simulink model "alfa_window_in_Ug"  (R2018b)
settings: Solver=VariableStepDiscrete  StartTime=0  StopTime=24*3600  MaxStep=1  RelTol=1e-3  EnableMultiTasking=on
libraries: carnot x5
settings Model: Creator=drhf  LastModifiedBy=drhf
settings DataIOCC: SaveFormat=Array  SignalLoggingSaveFormat=ModelDataLogs
settings OptimizationCC: ExpressionDepthLimit=2147483647  LifeSpan=inf
settings DebuggingCC: UnderspecifiedInitializationDetection=Classic  MergeDetectMultiDrivingBlocksExec=none  SolverPrmCheckMsg=warning  StateNameClashWarn=warning  SFUnexpectedBacktrackingDiag=warning  SFNoUnconditionalDefaultTransitionDiag=warning  SFExecutionAtInitializationDiag=none
settings HardwareCC: ProdBitPerPointer=32  ProdBitPerSizeT=32  ProdBitPerPtrDiffT=32  ProdLargestAtomicFloat=None  ProdIntDivRoundTo=Undefined  ProdEndianess=Unspecified  ProdWordSize=32  ProdHWDeviceType=32-bit Generic
settings ModelReferenceCC: PropagateSignalLabelsOutOfModel=off
settings SFSimCC: SimUseLocalCustomCode=off
settings RTWCC: RTWUseLocalCustomCode=off
settings CodeAppCC: StateflowObjectComments=on
settings GRTTargetCC: TargetLangStandard=C89/C90 (ANSI)  GeneratePreprocessorConditionals=Disable all  CombineOutputUpdateFcns=off  GRTInterface=on
settings ConfigComp: CovMetricSettings=dw  CovHtmlReporting=on  CovSaveCumulativeToWorkspaceVar=on  CovSaveSingleToWorkspaceVar=on  CovExternalEMLEnable=off

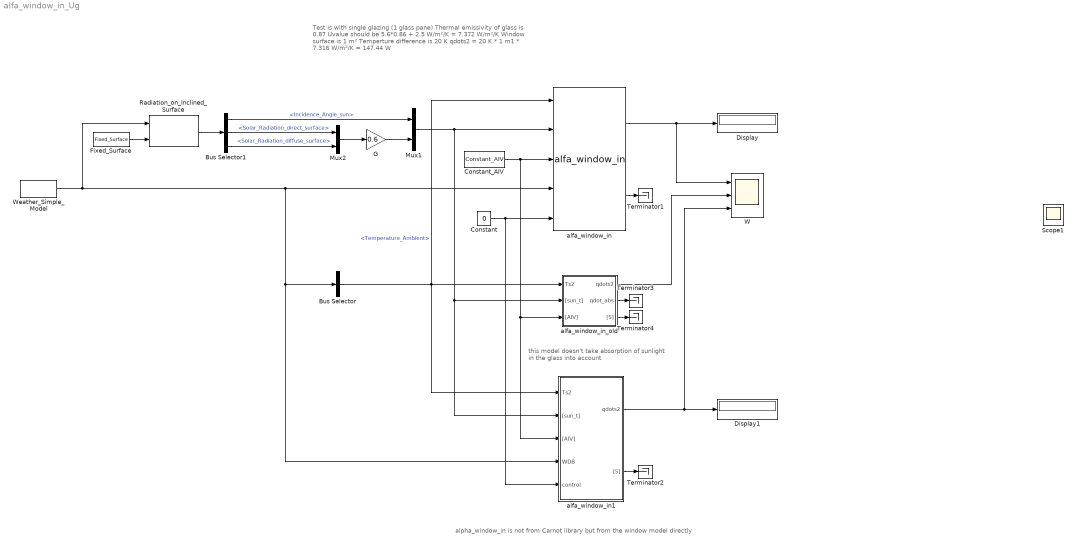
== system alfa_window_in_Ug ==
  note: this model doesn't take absorption
      | of sunlight in the glass into account
  note: Test is with single glazing (1 glass pane)
      | Thermal emissivity of glass is 0.87
      | Uvalue should be 5.6*0.86 + 2.5 W/m²/K = 7.372 W/m²/K
      | Window surface is 1 m²
      | Temperture difference is 20 K
      | qdots2 = 20 K * 1 m1 * 7.316 W/m²/K = 147.44 W
  note: alpha_window_in is not from Carnot library but from the window model directly
  Bus Selector : BusSelector  OutputSignals=Temperature_Ambient
  Bus Selector1 : BusSelector  OutputSignals=Incidence_Angle_sun,Solar_Radiation_direct_surface,Solar_Radiation_diffuse_surface
  Constant : Constant  Value=0
  Constant_AIV : carnot/Source/Ventilation/Constant_AIV  Tsens=20  Tcon=20  Trad=20  mw=0.012  mco=0.01  rhoair=1.2  cpair=1004  pair=100000  nair=0.5
      settings: SourceProductName=Carnot
  Display : Display
  Display1 : Display
  Fixed_Surface : carnot/Weather/Fixed_Surface  colangle=90  colazi=0  colrot=0
      settings: SourceProductName=Carnot
  G : Gain  Gain=0.6
  Mux1 : Mux  Inputs=2
  Mux2 : Mux  Inputs=2
  Radiation_on_Inclined_Surface : carnot/Weather/Radiation_on_Inclined_Surface  sky=Perez 1990  reflect=0.2
      settings: SourceProductName=Carnot
  Terminator{1..4} (4 alike) : Terminator
  W : Scope  NumInputPorts=3
  Weather_Simple_Model : carnot/Weather/Weather_Simple_Model  Ibn=900  Idg=100  tamb=0  deltaTsky=0  rh=50  precip="10e-3/24/3600           % 10 mm in 24 h"  cloud=0.125  p=1013e2  vw=0  wdir=270  lat=60  colangle=0  colazi=0  colrot=0
      settings: SourceProductName=Carnot
  alfa_window_in : carnot/Basic/Heat_Transfer/alfa_window_in  type_glazing=double glazing normal  gvalue=0.8  tauzero=0.9  emission_in=0.87  wallsurface=1  frame=0  numlayer=1  shad_type=No shading  tau_shad=0.01  bli_a=0.05  bli_b=1  bli_c=0.05  bli_d=0.05  bli_alpha=90  bli_refl=0.2
      settings: SourceProductName=Carnot
  alfa_window_in1 : Subsystem  mask(ALFA){}
      mask help:
      | Convective and radiative heat transfer at the INDOOR SURFACE OF A VERTICAL WINDOW with 1-4 layers (each 3 ... 8 mm thick).
      |
      | Ts  : temperature of window surface, °C,
      | [sun_t]  : sun data (incidence angle, direct and diffuse radiation
      |     at tilted window surface),
      | [AIV]  : conditions of zone node,
      | qdots  : specific heat flow into window construction, W/m^2,
      | [S]  : heat and air flow to zone node.
  alfa_window_in_old : Subsystem  mask(ALFA){gvalue=0.7, emission_in=0.87, wallsurface=1, frame=0.1, numlayer=2}
      mask prompts: gvalue "Energy transmission by sunlight (g-value) 0..1"; emission_in "Longwave emissivity (0..1)"; wallsurface "Surface of the window (with frame) in m²"; frame "Share of the frame on the surface (0...1)"; numlayer "Number of glass panes"
      mask help:
      | Convective and radiative heat transfer at the INDOOR SURFACE OF A VERTICAL WINDOW with 1-4 layers (each 3 ... 8 mm thick).
      |
      | Ts  : temperature of window surface, °C,
      | [sun_t]  : sun data (incidence angle, direct and diffuse radiation
      |     at tilted window surface),
      | [AIV]  : conditions of zone node,
      | qdots  : specific heat flow into window construction, W/m^2,
      | qdot_abs : specific irradiation absorption within window
      |     construction,  W/m^2,
      | [S]  : heat and air flow to zone node.
      mask Help: web(fullfile(path_carnot('help'),'alfa_window_in.html'),'-helpbrowser')
  Scope1 : Scope
  wires:
  alfa_window_in/1 -> Display/1, W/1
  Bus Selector/1 -> alfa_window_in/1, alfa_window_in1/1(Ts2), alfa_window_in_old/1(Ts2)  "<Temperature_Ambient>"
  Constant_AIV/1 -> alfa_window_in/3, alfa_window_in_old/3("[AIV]"), alfa_window_in1/3("[AIV]")
  Mux1/1 -> alfa_window_in1/2("[sun_t]"), alfa_window_in_old/2("[sun_t]"), alfa_window_in/2
  Weather_Simple_Model/1 -> Radiation_on_Inclined_Surface/1, Bus Selector/1, alfa_window_in1/4(WDB), alfa_window_in/4
  Constant/1 -> alfa_window_in1/5(control), alfa_window_in/5
  alfa_window_in_old/2(qdot_abs) -> Terminator3/1
  alfa_window_in_old/3("[S]") -> Terminator4/1
  alfa_window_in_old/1(qdots2) -> W/2
  Bus Selector1/1 -> Mux1/1  "<Incidence_Angle_sun>"
  Bus Selector1/3 -> Mux2/2  "<Solar_Radiation_diffuse_surface>"
  Radiation_on_Inclined_Surface/1 -> Bus Selector1/1
  Bus Selector1/2 -> Mux2/1  "<Solar_Radiation_direct_surface>"
  Mux2/1 -> G/1
  Fixed_Surface/1 -> Radiation_on_Inclined_Surface/2
  G/1 -> Mux1/2
  alfa_window_in/2 -> Terminator1/1
  alfa_window_in1/2("[S]") -> Terminator2/1
  alfa_window_in1/1(qdots2) -> Display1/1, W/3

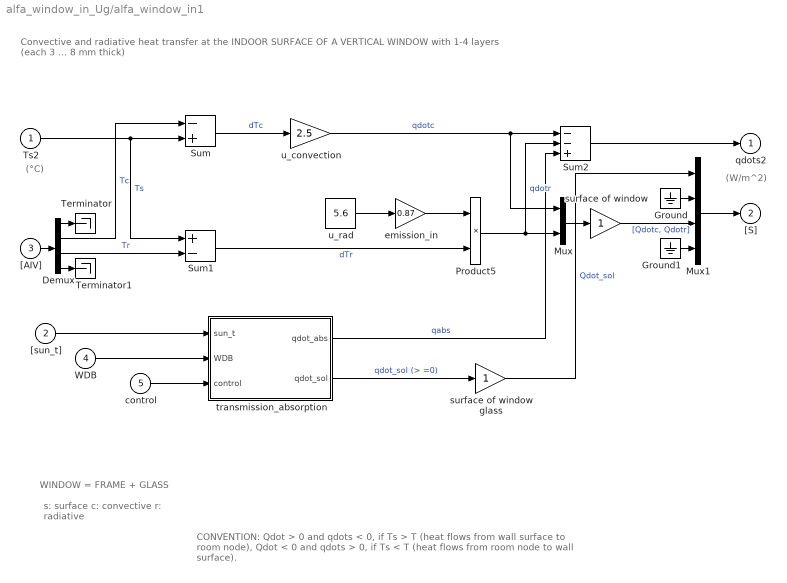
== system alfa_window_in_Ug/alfa_window_in1 ==
  note: (°C)
  note: Convective and radiative heat transfer at the INDOOR SURFACE OF A VERTICAL WINDOW
      | with 1-4 layers (each 3 ... 8 mm thick)
  note: WINDOW = FRAME + GLASS
  note: s: surface
      | c: convective
      | r: radiative
  note: CONVENTION:
      | Qdot > 0 and qdots < 0, if Ts > T (heat flows from wall surface to room node),
      | Qdot < 0 and qdots > 0, if Ts < T (heat flows from room node to wall surface).
  note: (W/m^2)
  Ts2 : Inport
  "[sun_t]" : Inport  Port=2
  "[AIV]" : Inport  Port=3
  WDB : Inport  Port=4
  control : Inport  Port=5
  Demux : Demux  Outputs=[1 1 1 6]
  Ground : Ground
  Ground1 : Ground
  Mux : Mux  Inputs=2
  Mux1 : Mux  Inputs=[1 5 2 5]
  Product5 : Product  SaturateOnIntegerOverflow=on  RndMeth=Zero  InputSameDT=on  OutDataTypeStr=Inherit: Same as first input
  Sum : Sum  Inputs=-+  SaturateOnIntegerOverflow=on  InputSameDT=on  OutDataTypeStr=Inherit: Same as first input
  Sum1 : Sum  Inputs=+-  SaturateOnIntegerOverflow=on  InputSameDT=on  OutDataTypeStr=Inherit: Same as first input
  Sum2 : Sum  Inputs=--+  SaturateOnIntegerOverflow=on  InputSameDT=on  OutDataTypeStr=Inherit: Same as first input
  Terminator : Terminator
  Terminator1 : Terminator
  emission_in : Gain  Gain=0.87  SaturateOnIntegerOverflow=on  OutDataTypeStr=Inherit: Same as input  ParamDataTypeStr=Inherit: Same as input
  surface of window : Gain  SaturateOnIntegerOverflow=on  OutDataTypeStr=Inherit: Same as input  ParamDataTypeStr=Inherit: Same as input
  surface of window glass : Gain  SaturateOnIntegerOverflow=on  OutDataTypeStr=Inherit: Same as input  ParamDataTypeStr=Inherit: Same as input
  transmission_absorption : Subsystem
  u_convection : Gain  Gain=2.5  SaturateOnIntegerOverflow=on  OutDataTypeStr=Inherit: Same as input  ParamDataTypeStr=Inherit: Same as input
  u_rad : Constant  Value=5.6
  qdots2 : Outport
  "[S]" : Outport  Port=2
  wires:
  control/1 -> transmission_absorption/3(control)
  WDB/1 -> transmission_absorption/2(WDB)
  transmission_absorption/1(qdot_abs) -> Sum2/3  "qabs"
  transmission_absorption/2(qdot_sol) -> surface of window glass/1  "qdot_sol (> =0)"
  Demux/3 -> Sum1/2  "Tr"
  Sum/1 -> u_convection/1  "dTc"
  Demux/2 -> Sum/1  "Tc"
  surface of window/1 -> Mux1/3  "[Qdotc, Qdotr]"
  surface of window glass/1 -> Mux1/1  "Qdot_sol"
  "[sun_t]"/1 -> transmission_absorption/1(sun_t)
  u_convection/1 -> Mux/1, Sum2/1  "qdotc"
  Product5/1 -> Sum2/2, Mux/2  "qdotr"
  Ts2/1 -> Sum1/1, Sum/2  "Ts"
  u_rad/1 -> emission_in/1
  Sum1/1 -> Product5/2  "dTr"
  emission_in/1 -> Product5/1
  Mux/1 -> surface of window/1
  Demux/1 -> Terminator/1
  "[AIV]"/1 -> Demux/1
  Demux/4 -> Terminator1/1
  Sum2/1 -> qdots2/1
  Mux1/1 -> "[S]"/1
  Ground/1 -> Mux1/2
  Ground1/1 -> Mux1/4

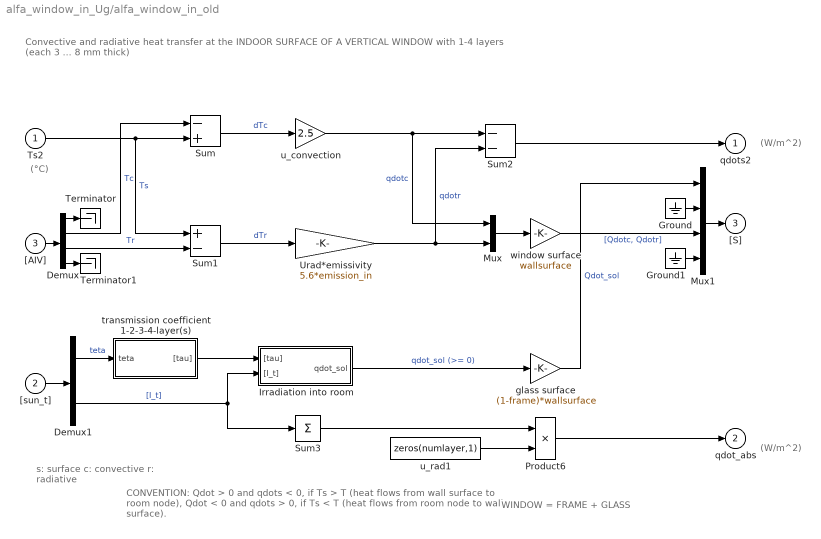
== system alfa_window_in_Ug/alfa_window_in_old ==
  note: (W/m^2)
  note: CONVENTION:
      | Qdot > 0 and qdots < 0, if Ts > T (heat flows from wall surface to room node),
      | Qdot < 0 and qdots > 0, if Ts < T (heat flows from room node to wall surface).
  note: s: surface
      | c: convective
      | r: radiative
  note: WINDOW = FRAME + GLASS
  note: (W/m^2)
  note: Convective and radiative heat transfer at the INDOOR SURFACE OF A VERTICAL WINDOW
      | with 1-4 layers (each 3 ... 8 mm thick)
  note: (°C)
  Ts2 : Inport
  "[sun_t]" : Inport  Port=2
  "[AIV]" : Inport  Port=3
  " glass surface" : Gain  Gain=(1-frame)*wallsurface  SaturateOnIntegerOverflow=on  OutDataTypeStr=Inherit: Same as input  ParamDataTypeStr=Inherit: Same as input
  Demux : Demux  Outputs=[1 1 1 6]
  Demux1 : Demux  Outputs=[1 2]
  Ground : Ground
  Ground1 : Ground
  Irradiation into room : Subsystem
  Mux : Mux  Inputs=2
  Mux1 : Mux  Inputs=[1 5 2 5]
  Product6 : Product  SaturateOnIntegerOverflow=on  InputSameDT=on  OutDataTypeStr=Inherit: Same as first input
  Sum : Sum  Inputs=-+  SaturateOnIntegerOverflow=on  InputSameDT=on  OutDataTypeStr=Inherit: Same as first input
  Sum1 : Sum  Inputs=+-  SaturateOnIntegerOverflow=on  InputSameDT=on  OutDataTypeStr=Inherit: Same as first input
  Sum2 : Sum  Inputs=--  SaturateOnIntegerOverflow=on  InputSameDT=on  OutDataTypeStr=Inherit: Same as first input
  Sum3 : Sum  Inputs=1  SaturateOnIntegerOverflow=on  InputSameDT=on  OutDataTypeStr=Inherit: Same as first input
  Terminator : Terminator
  Terminator1 : Terminator
  Urad*emissivity : Gain  Gain=5.6*emission_in  SaturateOnIntegerOverflow=on  OutDataTypeStr=Inherit: Same as input  ParamDataTypeStr=Inherit: Same as input
  transmission coefficient 1-2-3-4-layer(s) : Subsystem
  u_convection : Gain  Gain=2.5  SaturateOnIntegerOverflow=on  OutDataTypeStr=Inherit: Same as input  ParamDataTypeStr=Inherit: Same as input
  u_rad1 : Constant  Value=zeros(numlayer,1)
  window surface : Gain  Gain=wallsurface  SaturateOnIntegerOverflow=on  OutDataTypeStr=Inherit: Same as input  ParamDataTypeStr=Inherit: Same as input
  qdots2 : Outport
  qdot_abs : Outport  Port=2
  "[S]" : Outport  Port=3
  wires:
  Sum3/1 -> Product6/1
  Product6/1 -> qdot_abs/1
  Ground1/1 -> Mux1/4
  Ground/1 -> Mux1/2
  Mux1/1 -> "[S]"/1
  Sum2/1 -> qdots2/1
  Demux/4 -> Terminator1/1
  "[AIV]"/1 -> Demux/1
  Demux/1 -> Terminator/1
  Mux/1 -> window surface/1
  Sum1/1 -> Urad*emissivity/1  "dTr"
  Ts2/1 -> Sum/2, Sum1/1  "Ts"
  Urad*emissivity/1 -> Sum2/2, Mux/2  "qdotr"
  u_convection/1 -> Mux/1, Sum2/1  "qdotc"
  Irradiation into room/1(qdot_sol) -> " glass surface"/1  "qdot_sol (>= 0)"
  Demux1/1 -> transmission coefficient 1-2-3-4-layer(s)/1(teta)  "teta"
  "[sun_t]"/1 -> Demux1/1
  " glass surface"/1 -> Mux1/1  "Qdot_sol"
  window surface/1 -> Mux1/3  "[Qdotc, Qdotr]"
  Demux/2 -> Sum/1  "Tc"
  u_rad1/1 -> Product6/2
  Sum/1 -> u_convection/1  "dTc"
  Demux/3 -> Sum1/2  "Tr"
  Demux1/2 -> Irradiation into room/2("[I_t]"), Sum3/1  "[I_t]"
  transmission coefficient 1-2-3-4-layer(s)/1("[tau]") -> Irradiation into room/1("[tau]")

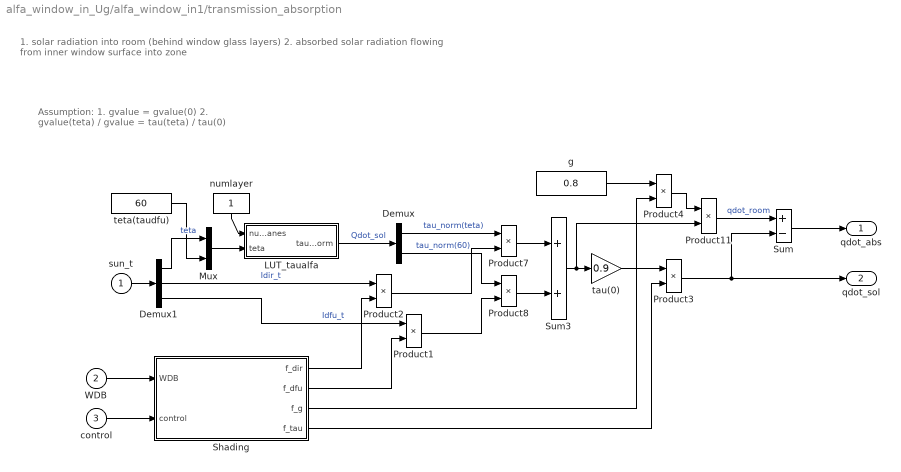
== system alfa_window_in_Ug/alfa_window_in1/transmission_absorption ==
  note: Assumption:
      | 1. gvalue = gvalue(0)
      | 2. gvalue(teta) / gvalue = tau(teta) / tau(0)
  note: 1. solar radiation into room (behind window glass layers)
      | 2. absorbed solar radiation flowing from inner window surface into zone
  sun_t : Inport
  WDB : Inport  Port=2
  control : Inport  Port=3
  Demux : Demux  Outputs=2
  Demux1 : Demux  Outputs=3
  LUT_taualfa : Subsystem  mask(LOOK UP TABLE){}
      mask help:
      | Normalized RADIATION TRANSMISSION COEFFICIENT of a window glass layer stack with 1, 2, 3 or 4 layers depending on the incidence angle.
      |
      | teta		: incidence angle = angle between surface normal and
      | 	                incidence direction, degree
      | numlayer	: number of layers within the window glass, [1,4].
      | tau		: transmission of glass layer stack, [0,1]
      |
      | NOTE: This block is defined for pane thickness between 3 and 6 mm.
  Mux : Mux  Inputs=2
  Product{1..4,7..8} (6 alike) : Product  SaturateOnIntegerOverflow=on  RndMeth=Zero  InputSameDT=on  OutDataTypeStr=Inherit: Same as first input
  Product11 : Product  Inputs=**  SaturateOnIntegerOverflow=on  RndMeth=Zero  InputSameDT=on  OutDataTypeStr=Inherit: Same as first input
  Shading : Subsystem
  Sum : Sum  Inputs=+-  SaturateOnIntegerOverflow=on  InputSameDT=on  OutDataTypeStr=Inherit: Same as first input
  Sum3 : Sum  SaturateOnIntegerOverflow=on  InputSameDT=on  OutDataTypeStr=Inherit: Same as first input
  g : Constant  Value=0.8
  numlayer : Constant
  tau(0) : Gain  Gain=0.9  SaturateOnIntegerOverflow=on  OutDataTypeStr=Inherit: Same as input  ParamDataTypeStr=Inherit: Same as input
  teta(taudfu) : Constant  Value=60
  qdot_abs : Outport
  qdot_sol : Outport  Port=2
  wires:
  control/1 -> Shading/2(control)
  WDB/1 -> Shading/1(WDB)
  Shading/3(f_g) -> Product4/2
  g/1 -> Product4/1
  Product4/1 -> Product11/1
  Shading/4(f_tau) -> Product3/2
  Shading/2(f_dfu) -> Product1/2
  Shading/1(f_dir) -> Product2/2
  Product2/1 -> Product7/2
  Demux1/2 -> Product2/1  "Idir_t"
  Product1/1 -> Product8/2
  Demux1/3 -> Product1/1  "Idfu_t"
  Product3/1 -> qdot_sol/1, Sum/2
  tau(0)/1 -> Product3/1
  sun_t/1 -> Demux1/1
  LUT_taualfa/1(tau_norm) -> Demux/1  "Qdot_sol"
  Demux/1 -> Product7/1  "tau_norm(teta)"
  Product7/1 -> Sum3/1
  Product8/1 -> Sum3/2
  Sum3/1 -> Product11/2, tau(0)/1
  Demux/2 -> Product8/1  "tau_norm(60)"
  Product11/1 -> Sum/1  "qdot_room"
  Sum/1 -> qdot_abs/1
  Demux1/1 -> Mux/1  "teta"
  teta(taudfu)/1 -> Mux/2
  numlayer/1 -> LUT_taualfa/1(numlpanes)
  Mux/1 -> LUT_taualfa/2(teta)

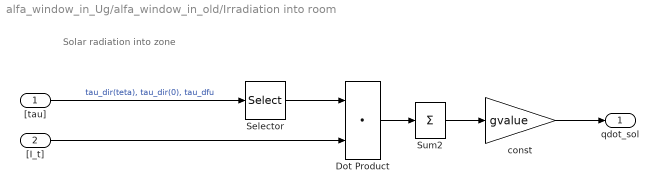
== system alfa_window_in_Ug/alfa_window_in_old/Irradiation into room ==
  note: Solar radiation into zone
  "[tau]" : Inport
  "[I_t]" : Inport  Port=2
  Dot Product : DotProduct  InputSameDT=on  OutDataTypeStr=Inherit: Inherit via internal rule
  Selector : Selector  InputPortWidth=3  IndexOptions=Index vector (dialog)  Indices=[1 3]  OutputSizes=1
  Sum2 : Sum  Inputs=1  SaturateOnIntegerOverflow=on  InputSameDT=on  OutDataTypeStr=Inherit: Same as first input
  const : Gain  Gain=gvalue  SaturateOnIntegerOverflow=on  OutDataTypeStr=Inherit: Same as input  ParamDataTypeStr=Inherit: Same as input
  qdot_sol : Outport
  wires:
  const/1 -> qdot_sol/1
  Sum2/1 -> const/1
  Dot Product/1 -> Sum2/1
  Selector/1 -> Dot Product/1
  "[tau]"/1 -> Selector/1  "tau_dir(teta), tau_dir(0), tau_dfu"
  "[I_t]"/1 -> Dot Product/2

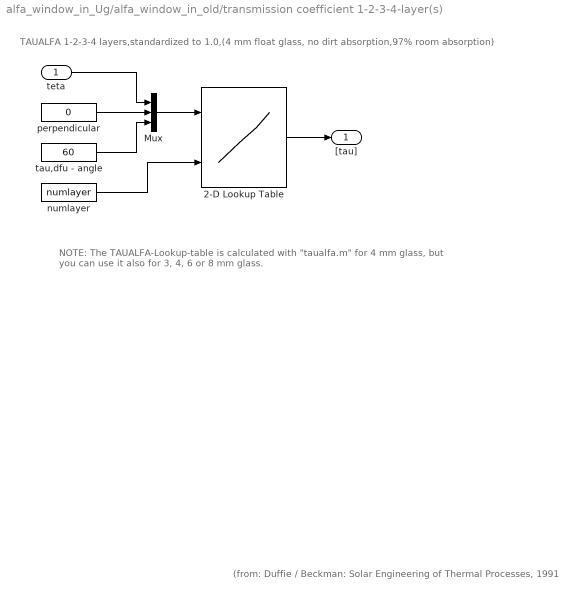
== system alfa_window_in_Ug/alfa_window_in_old/transmission coefficient 1-2-3-4-layer(s) ==
  note: NOTE: The TAUALFA-Lookup-table is calculated with "taualfa.m"
      | for 4 mm glass, but you can use it also for  3, 4, 6 or 8 mm glass.
  note: (from: Duffie / Beckman: Solar Engineering of Thermal Processes, 1991
  note: TAUALFA 1-2-3-4 layers,standardized to 1.0,(4 mm float glass, no dirt absorption,97% room absorption)
  teta : Inport
  2-D Lookup Table : Lookup_n-D  BreakpointsForDimension1=[0:10:90]  BreakpointsForDimension2=[1:4]  Table=[1.0000 1.0000 1.0000 1.0000; 0.9996 0.9991 0.9987 0.9983; 0.9979 0.9961 0.9945 0.9929; 0.9937 0.9894 0.9861 0.9836; 0.9839 0.9753 0.9704 0.9680; 0.9608 0.9438 0.9365 0.9361; 0.9061 0.8679 0.8484 0.8413; 0.7755 0.6821 0.6182 0.5717; 0.4807 0.3277 0.2324 0.1688; 0 0 0 0]  InternalRulePriority=Speed  RndMeth=Simplest  InputSameDT=on
  Mux : Mux  Inputs=3
  numlayer : Constant  Value=numlayer
  perpendicular : Constant  Value=0
  tau,dfu - angle : Constant  Value=60
  "[tau]" : Outport
  wires:
  2-D Lookup Table/1 -> "[tau]"/1
  numlayer/1 -> 2-D Lookup Table/2
  Mux/1 -> 2-D Lookup Table/1
  perpendicular/1 -> Mux/2
  tau,dfu - angle/1 -> Mux/3
  teta/1 -> Mux/1

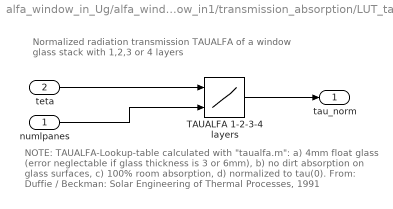
== system alfa_window_in_Ug/alfa_window_in1/transmission_absorption/LUT_taualfa ==
  note: NOTE:
      | TAUALFA-Lookup-table calculated with "taualfa.m":
      |   a) 4mm float glass (error neglectable if glass thickness is 3 or 6mm),
      |   b) no dirt absorption on glass surfaces,
      |   c) 100% room absorption,
      |   d) normalized to tau(0).
      |
      | From: Duffie / Beckman: Solar Engineering of Thermal Processes, 1991
  note: Normalized radiation transmission TAUALFA
      | of a window glass stack with 1,2,3 or 4 layers
  numlpanes : Inport
  teta : Inport  Port=2
  TAUALFA 1-2-3-4 layers : Lookup2D  RowIndex=[0:10:90]  ColumnIndex=[1:4]  Table="[1  1  1  1;.99955 .99912  .9987 .99827;.99787  .9961 .99449 .99298;.99364 .98941 .98618 .98366;.98364 .97519 .97041 .96824;.9601 .94337 .93638 .93624;.90423 .86634 .84734 .84064;.77129 .67843 .61507 .56891;.47436  .3235 .22952 .16682;0  0  0  0]"  SaturateOnIntegerOverflow=on  InputSameDT=on
  tau_norm : Outport
  wires:
  teta/1 -> TAUALFA 1-2-3-4 layers/1
  numlpanes/1 -> TAUALFA 1-2-3-4 layers/2
  TAUALFA 1-2-3-4 layers/1 -> tau_norm/1

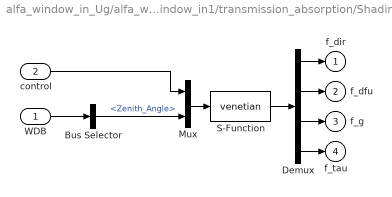
== system alfa_window_in_Ug/alfa_window_in1/transmission_absorption/Shading ==
  WDB : Inport
  control : Inport  Port=2
  Bus Selector : BusSelector  OutputSignals=Zenith_Angle
  Demux : Demux
  Mux : Mux  Inputs=2
  S-Function : S-Function  FunctionName=venetian  Parameters=0, 0, 0, 0, 0, 0, 1, 1, 0  SFunctionDeploymentMode=off  EnableBusSupport=off
  f_dir : Outport
  f_dfu : Outport  Port=2
  f_g : Outport  Port=3
  f_tau : Outport  Port=4
  wires:
  WDB/1 -> Bus Selector/1
  Bus Selector/1 -> Mux/2  "<Zenith_Angle>"
  control/1 -> Mux/1
  Mux/1 -> S-Function/1
  S-Function/1 -> Demux/1
  Demux/1 -> f_dir/1
  Demux/2 -> f_dfu/1
  Demux/3 -> f_g/1
  Demux/4 -> f_tau/1
